simulink model "nestedcbor"  (R2024b)
settings: Solver=VariableStepAuto  StartTime=0.0  StopTime=inf  RelTol=1e-3
libraries: simulink x1
settings Model: ModifiedByFormat=The MathWorks, Inc.  Creator=The MathWorks, Inc.  LastModifiedBy=The MathWorks, Inc.
settings SolverCC: AlgebraicLoopSolver=TrustRegion
settings DebuggingCC: UnconnectedInputMsg=warning  UnconnectedOutputMsg=warning  UnconnectedLineMsg=warning
settings ModelReferenceCC: EnableRefExpFcnMdlSchedulingChecks=on
settings RTWCC: GPUComputeCapability=3.5  DLArmComputeVersion=19.05

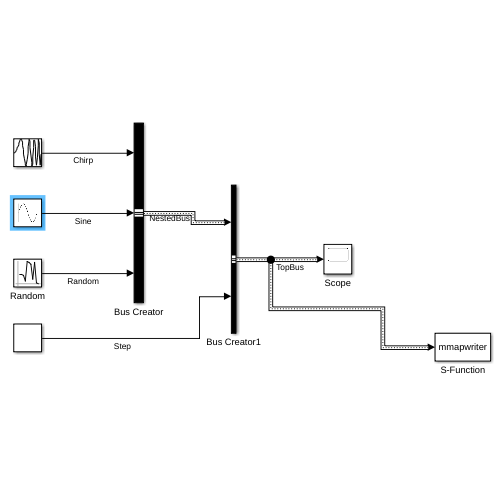
[thumbnail: Simulink's stored preview of the top-level diagram]
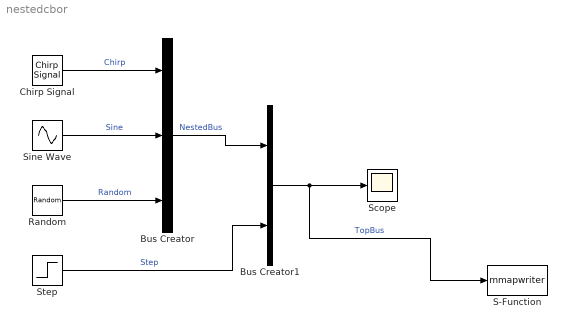
== system nestedcbor ==
  Bus Creator : BusCreator  Inputs=3  OutDataTypeStr=Bus: NestedBus  NonVirtualBus=on
      settings: InheritFromInputs=off
  Bus Creator1 : BusCreator  Inputs=2  OutDataTypeStr=Bus: TopBus  NonVirtualBus=on
      settings: InheritFromInputs=off
  Chirp Signal : simulink/Sources/Chirp Signal  f1=0.1  T=100  f2=1
  Random : RandomNumber  SampleTime=0
  S-Function : S-Function  FunctionName=mmapwriter  Parameters='TopBus', 'Testing'  SFunctionDeploymentMode=off  EnableBusSupport=off
  Scope : Scope
  Sine Wave : Sin  SampleTime=0
  Step : Step  SampleTime=0
  wires:
  Sine Wave/1 -> Bus Creator/2  "Sine"
  Bus Creator/1 -> Bus Creator1/1  "NestedBus"
  Chirp Signal/1 -> Bus Creator/1  "Chirp"
  Step/1 -> Bus Creator1/2  "Step"
  Bus Creator1/1 -> S-Function/1, Scope/1  "TopBus"
  Random/1 -> Bus Creator/3  "Random"
